simulink model "ECS_Lidar_sensor"  (R2025a)
settings: Solver=ode45  StartTime=0.0  StopTime=3600  RelTol=1e-3
libraries: fl_lib x15, nesl_utility x8
settings Model: Creator=Piyusha  LastModifiedBy=Piyusha
settings SolverCC: ZeroCrossAlgorithm=Adaptive

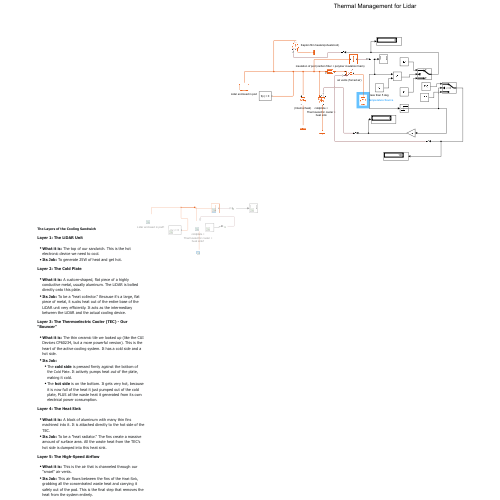
[thumbnail: Simulink's stored preview of the top-level diagram]
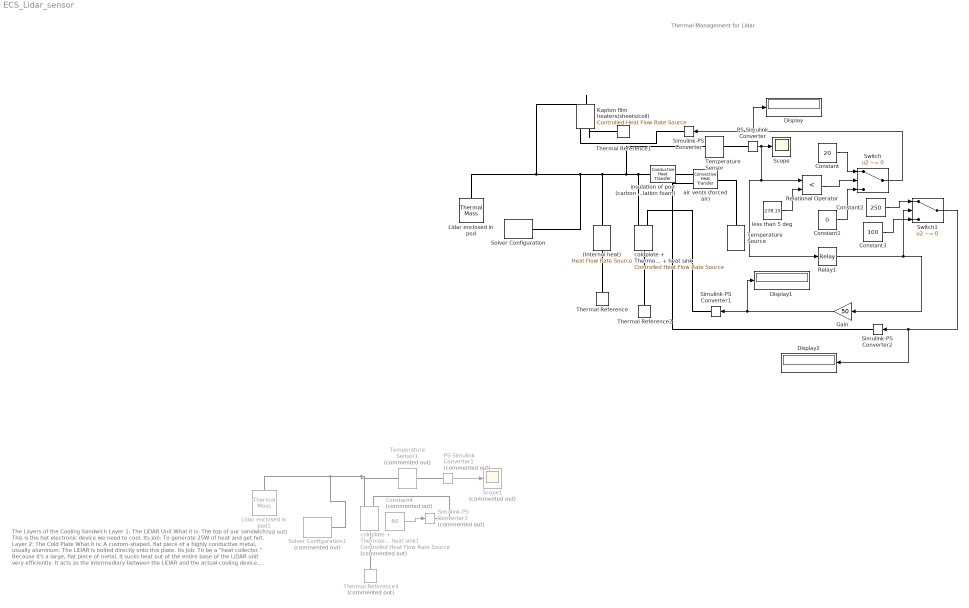
== system ECS_Lidar_sensor ==
  note: The Layers of the Cooling Sandwich
      | Layer 1: The LiDAR Unit
      | What it is: The top of our sandwich. This is the hot electronic device we need to cool.
      | Its Job: To generate 25W of heat and get hot.
      | Layer 2: The Cold Plate
      | What it is: A custom-shaped, flat piece of a highly conductive metal, usually aluminum. The LiDAR is bolted directly onto this plate.
      | Its Job: To be a "heat collector." Because it's a large, flat piece of metal, it sucks heat out of the entire base of the LiDAR unit very efficiently. It acts as the intermediary between the LiDAR and the actual cooling device.
      | Layer 3: The Thermoelectric Cooler (TEC) - Our "Bouncer"
      | What it is: The thin ceramic tile we looked up (like the CUI Devices CP60234, but a more powerful version). This is the heart of the active cooling system. It has a cold side and a hot side.
      | Its Job: The cold side is pressed firmly against the bottom of the Cold Plate . It actively pumps heat out of the plate, making it cold.
      | The hot side is on the bottom. It gets very hot, because it is now full of the heat it just pumped out of the cold plate, PLUS all the waste heat it generated from its own electrical power consumption.
      |
      | Layer 4: The Heat Sink
      | What it is: A block of aluminum with many thin fins machined into it. It is attached directly to the hot side of the TEC.
      | Its Job: To be a "heat radiator." The fins create a massive amount of surface area. All the waste heat from the TEC's hot side is dumped into this heat sink.
      | Layer 5: The High-Speed Airflow
      | What it is: This is the air that is channeled through our "smart" air vents.
      | Its Job: This air flows between the fins of the Heat Sink , grabbing all the concentrated waste heat and carrying it safely out of the pod. This is the final step that removes the heat from the system entirely.
  note: Thermal Management for Lidar
  (Internal heat) : fl_lib/Thermal/Thermal Sources/Heat Flow Rate Source  heat_flow=25 W
      settings: InternalSimscapePortConfiguration="{\"Bottom\":[],\"Left\":[{\"id\":\"B\",\"label\":\"B\",\"type\":\"foundation.thermal.thermal\"}],\"Right\":[{\"id\":\"A\",\"label\":\"A\",\"type\":\"foundation.thermal.thermal\"}],\"Top\":[]}"
  Constant : Constant  Value=20
  Constant1 : Constant  Value=0
  Constant2 : Constant  Value=250
  Constant3 : Constant  Value=100
  Constant4 : Constant  Commented=on  Value=60
  Display : Display
  Display1 : Display
  Display2 : Display
  Gain : Gain  Gain=50
  Kapton film heaters(sheets/coil) : fl_lib/Thermal/Thermal Sources/Controlled Heat Flow Rate Source
  Lidar enclosed in pod : fl_lib/Thermal/Thermal Elements/Thermal Mass  mass_type=foundation.enum.constant_variable.constant  mass=4.1 kg  sp_heat=900 J/(K*kg)  mass_min=1e-6 kg  num_ports=foundation.enum.numPorts2.one  m_specify=off  m_priority=High  m=1 kg  m_nominal_specify=off  m_nominal_value=1  m_nominal_unit=kg  T_specify=on  T_priority=High  T=45 degC  T_nominal_specify=off  T_nominal_value=1  T_nominal_unit=K  Q_specify=off  Q_priority=None  Q=0 W  Q_nominal_specify=off  Q_nominal_value=1  Q_nominal_unit=W
  Lidar enclosed in pod1 : fl_lib/Thermal/Thermal Elements/Thermal Mass  Commented=on  mass_type=foundation.enum.constant_variable.constant  mass=4.1 kg  sp_heat=900 J/(K*kg)  mass_min=1e-6 kg  num_ports=foundation.enum.numPorts2.one  m_specify=off  m_priority=High  m=1 kg  m_nominal_specify=off  m_nominal_value=1  m_nominal_unit=kg  T_specify=on  T_priority=High  T=20 degC  T_nominal_specify=off  T_nominal_value=1  T_nominal_unit=K  Q_specify=off  Q_priority=None  Q=0 W  Q_nominal_specify=off  Q_nominal_value=1  Q_nominal_unit=W
  PS-Simulink Converter : nesl_utility/PS-Simulink Converter  PhysicalDomain=network_engine_domain  SubClassName=ps_output  LeftPortType=input  RightPortType=output  PseudoPeriodic=off  Frequencies=[]  VectorFormat=inherit  Unit=K  AffineConversion=off
  PS-Simulink Converter1 : nesl_utility/PS-Simulink Converter  Commented=on  PhysicalDomain=network_engine_domain  SubClassName=ps_output  LeftPortType=input  RightPortType=output  PseudoPeriodic=off  Frequencies=[]  VectorFormat=inherit  Unit=K  AffineConversion=off
  Relational Operator : RelationalOperator  Operator=<  OutDataTypeStr=boolean  RndMeth=Simplest  InputSameDT=off
  Relay1 : Relay  OnSwitchValue=308.15  OffSwitchValue=307.15
  Scope : Scope
      settings: ActiveDisplayYMinimum=253.95851423403107  ActiveDisplayYMaximum=353.06995549291725
  Scope1 : Scope  Commented=on
      settings: ActiveDisplayYMinimum=266.52257904492308  ActiveDisplayYMaximum=296.4024695054996
  Simulink-PS Converter : nesl_utility/Simulink-PS Converter  PhysicalDomain=network_engine_domain  SubClassName=ps_input  LeftPortType=input  RightPortType=output  PseudoPeriodic=off  Frequencies=[]  NoiseDistribution=none  NoiseParameters=[]  Unit=W  AffineConversion=off  FilteringAndDerivatives=filter  SimscapeFilterOrder=1  InputFilterTimeConstant=0.001  UdotUserProvided=0
  Simulink-PS Converter1 : nesl_utility/Simulink-PS Converter  PhysicalDomain=network_engine_domain  SubClassName=ps_input  LeftPortType=input  RightPortType=output  PseudoPeriodic=off  Frequencies=[]  NoiseDistribution=none  NoiseParameters=[]  Unit=W  AffineConversion=off  FilteringAndDerivatives=filter  SimscapeFilterOrder=1  InputFilterTimeConstant=0.001  UdotUserProvided=0
  Simulink-PS Converter2 : nesl_utility/Simulink-PS Converter  PhysicalDomain=network_engine_domain  SubClassName=ps_input  LeftPortType=input  RightPortType=output  PseudoPeriodic=off  Frequencies=[]  NoiseDistribution=none  NoiseParameters=[]  Unit=W/(K*m^2)  AffineConversion=off  FilteringAndDerivatives=filter  SimscapeFilterOrder=1  InputFilterTimeConstant=0.001  UdotUserProvided=0
  Simulink-PS Converter3 : nesl_utility/Simulink-PS Converter  Commented=on  PhysicalDomain=network_engine_domain  SubClassName=ps_input  LeftPortType=input  RightPortType=output  PseudoPeriodic=off  Frequencies=[]  NoiseDistribution=none  NoiseParameters=[]  Unit=1  AffineConversion=off  FilteringAndDerivatives=provide  SimscapeFilterOrder=1  InputFilterTimeConstant=0.001  UdotUserProvided=0
  Solver Configuration : nesl_utility/Solver Configuration  PhysicalDomain=network_engine_domain  SubClassName=solver  LeftPortType=input  RightPortType=generic  Tones=[]  Harmonics=[]  SimulateNoise=off  Profile=off  UseLocalSampling=off  EnableSwitchedLinearOptims=on  FrequencyDomain=off  UseCCode=off  RelTol=0.001  AbsTol=0.001  MinStep=1e-09  ToWorkspace=off  RevertToSquareIcSolve=off  NumHomotopyIterations=100  PhasorMode=off  PhasorModeNumHarmonics=1  ConsistencySolver=NEWTON_XTOL_AFTER_FTOL  IndexReductionMethod=DerivativeReplacement  DoDC=off  ResidualTolerance=1e-09  ConsistencyTolSource=GLOBAL  ConsistencyAbsTol=0.001  ConsistencyRelTol=0.001  ConsistencyTolFactor=0.001  UseLocalSolver=off  LocalSolverChoice=NE_BACKWARD_EULER_ADVANCER  ResolveIndetEquations=on  FunctionEvalNumThread=1  LocalSolverSampleTime=0.001  DoFixedCost=off  MaxNonlinIter=3  MaxModeIter=2  ComputeImpulses=off  ImpulseIterations=2  LinearAlgebra=auto  LinearAlgebraNumThread=0  EquationFormulation=NE_TIME_EF  DelaysMemoryBudget=1024  AutomaticFiltering=on  FilteringTimeConstant=0.001  PartitionStorageMethod=AS_NEEDED  PartitionMemoryBudget=1024  PartitionMethod=ROBUST  MultibodyUseLocalSolver=off  MultibodyLocalSolverChoice=ODE1  MultibodyLocalSolverSampleTime=0.001
  Solver Configuration1 : nesl_utility/Solver Configuration  Commented=on  PhysicalDomain=network_engine_domain  SubClassName=solver  LeftPortType=input  RightPortType=generic  Tones=[]  Harmonics=[]  SimulateNoise=off  Profile=off  UseLocalSampling=off  EnableSwitchedLinearOptims=on  FrequencyDomain=off  UseCCode=off  RelTol=0.001  AbsTol=0.001  MinStep=1e-09  ToWorkspace=off  RevertToSquareIcSolve=off  NumHomotopyIterations=100  PhasorMode=off  PhasorModeNumHarmonics=1  ConsistencySolver=NEWTON_XTOL_AFTER_FTOL  IndexReductionMethod=DerivativeReplacement  DoDC=off  ResidualTolerance=1e-09  ConsistencyTolSource=GLOBAL  ConsistencyAbsTol=0.001  ConsistencyRelTol=0.001  ConsistencyTolFactor=0.001  UseLocalSolver=off  LocalSolverChoice=NE_BACKWARD_EULER_ADVANCER  ResolveIndetEquations=on  FunctionEvalNumThread=1  LocalSolverSampleTime=0.001  DoFixedCost=off  MaxNonlinIter=3  MaxModeIter=2  ComputeImpulses=off  ImpulseIterations=2  LinearAlgebra=auto  LinearAlgebraNumThread=0  EquationFormulation=NE_TIME_EF  DelaysMemoryBudget=1024  AutomaticFiltering=on  FilteringTimeConstant=0.001  PartitionStorageMethod=AS_NEEDED  PartitionMemoryBudget=1024  PartitionMethod=ROBUST  MultibodyUseLocalSolver=off  MultibodyLocalSolverChoice=ODE1  MultibodyLocalSolverSampleTime=0.001
  Switch : Switch  Criteria=u2 ~= 0  SaturateOnIntegerOverflow=off  InputSameDT=off
  Switch1 : Switch  Criteria=u2 ~= 0  SaturateOnIntegerOverflow=off  InputSameDT=off
  Temperature Sensor : fl_lib/Thermal/Thermal Sensors/Temperature Sensor  temperature_measure=foundation.enum.MeasurementReference.absolute
      settings: InternalSimscapePortConfiguration="{\"Bottom\":[],\"Left\":[{\"id\":\"A\",\"label\":\"A\",\"type\":\"foundation.thermal.thermal\"}],\"Right\":[{\"id\":\"T\",\"label\":\"T\",\"type\":\"output\"}],\"Top\":[]}"
  Temperature Sensor1 : fl_lib/Thermal/Thermal Sensors/Temperature Sensor  Commented=on  temperature_measure=foundation.enum.MeasurementReference.absolute
      settings: InternalSimscapePortConfiguration="{\"Bottom\":[],\"Left\":[{\"id\":\"A\",\"label\":\"A\",\"type\":\"foundation.thermal.thermal\"}],\"Right\":[{\"id\":\"T\",\"label\":\"T\",\"type\":\"output\"}],\"Top\":[]}"
  Temperature Source : fl_lib/Thermal/Thermal Sources/Temperature Source  temperature=45 degC
  Thermal Reference : fl_lib/Thermal/Thermal Elements/Thermal Reference
  Thermal Reference1 : fl_lib/Thermal/Thermal Elements/Thermal Reference
  Thermal Reference2 : fl_lib/Thermal/Thermal Elements/Thermal Reference
  Thermal Reference3 : fl_lib/Thermal/Thermal Elements/Thermal Reference  Commented=on
  air vents (forced air) : fl_lib/Thermal/Thermal Elements/Convective Heat Transfer  thermal_type=foundation.enum.constant_variable.variable  area=0.2 m^2  heat_tr_coeff=100 W/(K*m^2)  min_heat_tr_coeff=1e-3 W/(K*m^2)  T_specify=off  T_priority=None  T=0 K  T_nominal_specify=off  T_nominal_value=1  T_nominal_unit=K  Q_specify=off  Q_priority=None  Q=0 W  Q_nominal_specify=off  Q_nominal_value=1  Q_nominal_unit=W
      settings: InternalSimscapePortConfiguration="{\"Bottom\":[],\"Left\":[{\"id\":\"A\",\"label\":\"A\",\"type\":\"foundation.thermal.thermal\"},{\"id\":\"var_heat_tr_coeff\",\"label\":\"K\",\"type\":\"input\"}],\"Right\":[{\"id\":\"B\",\"label\":\"B\",\"type\":\"foundation.thermal.thermal\"}],\"Top\":[]}"
  coldplate + Thermoelectric cooler + heat sink : fl_lib/Thermal/Thermal Sources/Controlled Heat Flow Rate Source
  coldplate + Thermoelectric cooler + heat sink1 : fl_lib/Thermal/Thermal Sources/Controlled Heat Flow Rate Source  Commented=on
  insulation of pod (carbon fiber + polymer insulation foam) : fl_lib/Thermal/Thermal Elements/Conductive Heat Transfer  thermal_type=foundation.enum.ConstantVariableTabulated.Constant  wall_geometry=foundation.enum.ConductionWallGeometry.Planar  area=0.2 m^2  thickness=0.01 m  d_in=0.05 m  d_out=0.1 m  L=1 m  th_cond_min=10 W/(K*m)  th_cond=0.04 W/(K*m)  th_cond_TLU=[413, 401, 392, 383, 371, 357, 342] W/(K*m)  temp_TLU=[200, 273, 400, 600, 800, 1000, 1200] K  T_specify=off  T_priority=None  T=0 K  T_nominal_specify=off  T_nominal_value=1  T_nominal_unit=K  Q_specify=off  Q_priority=None  Q=0 W  Q_nominal_specify=off  Q_nominal_value=1  Q_nominal_unit=W
  less than 5 deg : Constant  Value=278.15
  wires:
  Switch/1 -> Display/1, Simulink-PS Converter/1
  PS-Simulink Converter/1 -> Relay1/1, Relational Operator/1, Scope/1
  Relay1/1 -> Switch1/2, Gain/1
  Constant/1 -> Switch/1
  Constant1/1 -> Switch/3
  less than 5 deg/1 -> Relational Operator/2
  Relational Operator/1 -> Switch/2
  Constant2/1 -> Switch1/1
  Constant3/1 -> Switch1/3
  Switch1/1 -> Simulink-PS Converter2/1, Display2/1
  Gain/1 -> Display1/1, Simulink-PS Converter1/1
  PS-Simulink Converter1/1 -> Scope1/1
  Constant4/1 -> Simulink-PS Converter3/1
  connections:
  Temperature Source/LConn1 -- air vents (forced air)/RConn1
  PS-Simulink Converter/LConn1 -- Temperature Sensor/RConn1
  (Internal heat)/RConn1 -- Thermal Reference/LConn1
  Kapton film heaters(sheets/coil)/RConn2 -- Thermal Reference1/LConn1
  Simulink-PS Converter/RConn1 -- Kapton film heaters(sheets/coil)/RConn1
  Thermal Reference2/LConn1 -- coldplate + Thermoelectric cooler + heat sink/LConn1
  Simulink-PS Converter1/RConn1 -- coldplate + Thermoelectric cooler + heat sink/RConn1
  Simulink-PS Converter2/RConn1 -- air vents (forced air)/LConn2
  Lidar enclosed in pod1/LConn1 -- Solver Configuration1/RConn1 -- Temperature Sensor1/LConn1 -- coldplate + Thermoelectric cooler + heat sink1/RConn2
  Thermal Reference3/LConn1 -- coldplate + Thermoelectric cooler + heat sink1/LConn1
  Temperature Sensor1/RConn1 -- PS-Simulink Converter1/LConn1
  Simulink-PS Converter3/RConn1 -- coldplate + Thermoelectric cooler + heat sink1/RConn1
  Kapton film heaters(sheets/coil)/LConn1 -- Temperature Sensor/LConn1 -- insulation of pod (carbon fiber + polymer insulation foam)/RConn1 -- coldplate + Thermoelectric cooler + heat sink/RConn2 -- (Internal heat)/LConn1 -- Solver Configuration/RConn1 -- Lidar enclosed in pod/LConn1
  air vents (forced air)/LConn1 -- insulation of pod (carbon fiber + polymer insulation foam)/LConn1
